simulink model "variant1"  (R2018a)
settings: Solver=VariableStepAuto  StartTime=0.0  StopTime=10.0  RelTol=1e-3
undefined symbols (not defined in the file or in its folder): gray
libraries: simulink x4, visionstatistics x2, visiontransforms x1
settings Model: Creator=Farwa  LastModifiedBy=Farwa

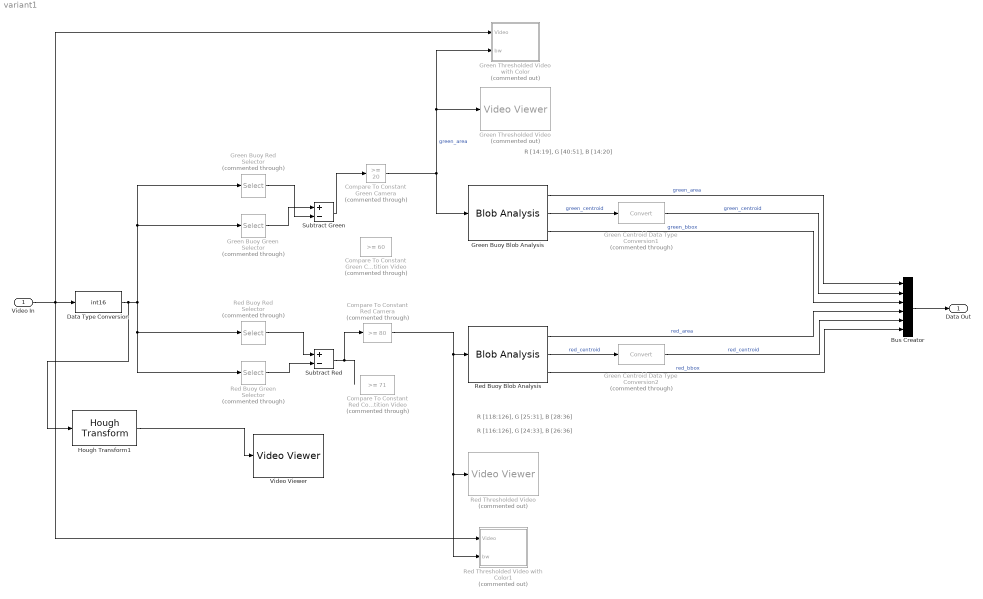
== system variant1 ==
  note: R [118:126], G [25:31], B [28:36]
  note: R [116:126], G [24:33], B [26:36]
  note: R [14:19], G [40:51], B [14:20]
  Video In : Inport
  Bus Creator : BusCreator  Inputs=6
  Compare To Constant Green Camera : simulink/Logic and Bit Operations/Compare To Constant  Commented=through  relop=>=  const=20  OutDataTypeStr=boolean
  Compare To Constant Green Competition Video : simulink/Logic and Bit Operations/Compare To Constant  Commented=through  relop=>=  const=60  OutDataTypeStr=boolean
  Compare To Constant Red Camera : simulink/Logic and Bit Operations/Compare To Constant  Commented=through  relop=>=  const=80  OutDataTypeStr=boolean
  Compare To Constant Red Competition Video : simulink/Logic and Bit Operations/Compare To Constant  Commented=through  relop=>=  const=71  OutDataTypeStr=boolean
  Data Type Conversion : DataTypeConversion  OutDataTypeStr=int16
  Green Buoy Blob Analysis : visionstatistics/Blob Analysis  Tag=vipblks_row_conv  area=on  centroid=on  bBox=on  majorAxis=off  minorAxis=off  angle=off  eccentricity=off  equivDiameterSq=off  extent=off  perimeter=off  maxBlobs=4  warnIfNumBlobsExceeded=off  isCount=off  useMinArea=on  minArea=40  useMaxArea=off  maxArea=100  excludeBorderBlob=off  outDT=single  isOutVarDim=off  isFill=on  fillValues=-1  conn=8  isLabel=off  outputMode=Binary point scaling  outputWordLength=32  outputFracLength=16  firstCoeffMode=Binary point scaling  firstCoeffWordLength=16  firstCoeffFracLength=14  secondCoeffMode=Binary point scaling  secondCoeffWordLength=32  secondCoeffFracLength=16  accumMode=Binary point scaling  accumWordLength=32  accumFracLength=0  prodOutputMode=Binary point scaling  prodOutputWordLength=32  prodOutputFracLength=16  roundingMode=Floor  overflowMode=off
      settings: SourceProductName=Computer Vision System Toolbox
  Green Buoy Green Selector : Selector  Commented=through  NumberOfDimensions=3  InputPortWidth=3  IndexOptions=Select all,Select all,Index vector (dialog)  Indices=[1 3],1,2  OutputSizes=1,1,1
  Green Buoy Red Selector : Selector  Commented=through  NumberOfDimensions=3  InputPortWidth=3  IndexOptions=Select all,Select all,Index vector (dialog)  Indices=[1 3],1,1  OutputSizes=1,1,1
  Green Centroid Data Type Conversion1 : DataTypeConversion  Commented=through
  Green Centroid Data Type Conversion2 : DataTypeConversion  Commented=through
  Green Thresholded Video : VideoViewer  Commented=on  colormapValue=gray(256)  FigPos=[1107 745 758 524]
  Green Thresholded Video with Color : Subsystem  Commented=on
  Hough Transform1 : visiontransforms/Hough Transform  theta_res=pi/180  rho_res=1  out_theta_rho=off  outdtmode=double  firstCoeffMode=Binary point scaling  firstCoeffWordLength=16  firstCoeffFracLength=14  secondCoeffMode=Binary point scaling  secondCoeffWordLength=32  secondCoeffFracLength=16  outputMode=Binary point scaling  outputWordLength=16  outputFracLength=0  accumMode=Binary point scaling  accumWordLength=32  accumFracLength=20  prodOutputMode=Binary point scaling  prodOutputWordLength=32  prodOutputFracLength=20  memoryMode=Binary point scaling  memoryWordLength=32  memoryFracLength=16  roundingMode=Nearest  overflowMode=on
      settings: SourceProductName=Computer Vision System Toolbox  SourceProductBaseCode=VP
  Red Buoy Blob Analysis : visionstatistics/Blob Analysis  Tag=vipblks_row_conv  area=on  centroid=on  bBox=on  majorAxis=off  minorAxis=off  angle=off  eccentricity=off  equivDiameterSq=off  extent=off  perimeter=off  maxBlobs=4  warnIfNumBlobsExceeded=off  isCount=off  useMinArea=on  minArea=20  useMaxArea=off  maxArea=100  excludeBorderBlob=off  outDT=double  isOutVarDim=off  isFill=on  fillValues=-1  conn=8  isLabel=off  outputMode=Binary point scaling  outputWordLength=32  outputFracLength=16  firstCoeffMode=Binary point scaling  firstCoeffWordLength=16  firstCoeffFracLength=14  secondCoeffMode=Binary point scaling  secondCoeffWordLength=32  secondCoeffFracLength=16  accumMode=Binary point scaling  accumWordLength=32  accumFracLength=0  prodOutputMode=Binary point scaling  prodOutputWordLength=32  prodOutputFracLength=16  roundingMode=Floor  overflowMode=off
      settings: SourceProductName=Computer Vision System Toolbox
  Red Buoy Green Selector : Selector  Commented=through  NumberOfDimensions=3  InputPortWidth=3  IndexOptions=Select all,Select all,Index vector (dialog)  Indices=[1 3],1,2  OutputSizes=1,1,1
  Red Buoy Red Selector : Selector  Commented=through  NumberOfDimensions=3  InputPortWidth=3  IndexOptions=Select all,Select all,Index vector (dialog)  Indices=[1 3],1,1  OutputSizes=1,1,1
  Red Thresholded Video : VideoViewer  Commented=on  colormapValue=gray(256)  FigPos=[1008 1320 758 524]
  Red Thresholded Video with Color1 : Subsystem  Commented=on
  Subtract Green : Sum  Inputs=+-  OutDataTypeStr=Inherit: Same as first input
  Subtract Red : Sum  Inputs=+-  OutDataTypeStr=Inherit: Same as first input
  Video Viewer : VideoViewer  FigPos=[431 511 418 304]
  Data Out : Outport
  wires:
  Green Buoy Blob Analysis/2 -> Green Centroid Data Type Conversion1/1  "green_centroid"
  Green Centroid Data Type Conversion1/1 -> Bus Creator/2  "green_centroid"
  Red Buoy Blob Analysis/1 -> Bus Creator/4  "red_area"
  Bus Creator/1 -> Data Out/1
  Red Buoy Green Selector/1 -> Subtract Red/2
  Green Buoy Blob Analysis/3 -> Bus Creator/3  "green_bbox"
  Red Buoy Blob Analysis/3 -> Bus Creator/6  "red_bbox"
  Compare To Constant Green Camera/1 -> Green Buoy Blob Analysis/1, Green Thresholded Video with Color/2(bw), Green Thresholded Video/1  "green_area"
  Subtract Green/1 -> Compare To Constant Green Camera/1
  Video In/1 -> Data Type Conversion/1, Green Thresholded Video with Color/1(Video), Red Thresholded Video with Color1/1(Video)
  Green Buoy Blob Analysis/1 -> Bus Creator/1  "green_area"
  Green Buoy Green Selector/1 -> Subtract Green/1
  Hough Transform1/1 -> Video Viewer/1
  Green Buoy Red Selector/1 -> Subtract Green/2
  Red Buoy Blob Analysis/2 -> Green Centroid Data Type Conversion2/1  "red_centroid"
  Red Buoy Red Selector/1 -> Subtract Red/1
  Data Type Conversion/1 -> Hough Transform1/1, Red Buoy Green Selector/1, Red Buoy Red Selector/1, Green Buoy Red Selector/1, Green Buoy Green Selector/1
  Green Centroid Data Type Conversion2/1 -> Bus Creator/5  "red_centroid"
  Compare To Constant Red Camera/1 -> Red Thresholded Video with Color1/2(bw), Red Thresholded Video/1, Red Buoy Blob Analysis/1
  Subtract Red/1 -> Compare To Constant Red Camera/1

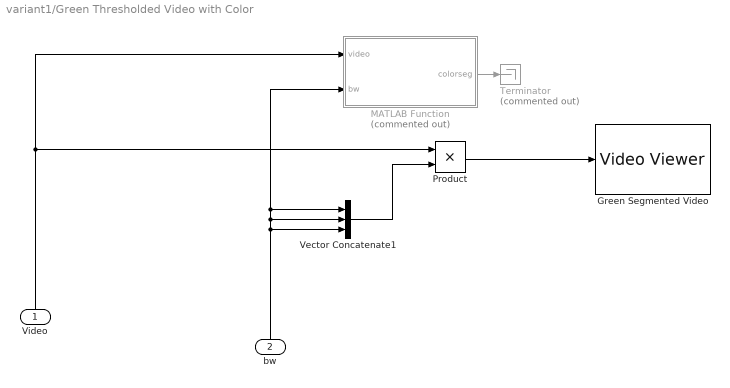
== system variant1/Green Thresholded Video with Color ==
  Video : Inport
  bw : Inport  Port=2
  "Green Segmented Video " : VideoViewer  colormapValue=gray(256)  FigPos=[1034 644 758 524]
  MATLAB Function : MATLAB Function  Commented=on  TreatAsAtomicUnit=on
  Product : Product
  Terminator : Terminator  Commented=on
  Vector Concatenate1 : Concatenate  NumInputs=3  Mode=Multidimensional array  ConcatenateDimension=3
  wires:
  bw/1 -> MATLAB Function/2(bw), Vector Concatenate1/1, Vector Concatenate1/2, Vector Concatenate1/3
  MATLAB Function/1(colorseg) -> Terminator/1
  Video/1 -> Product/1, MATLAB Function/1(video)
  Product/1 -> "Green Segmented Video "/1
  Vector Concatenate1/1 -> Product/2

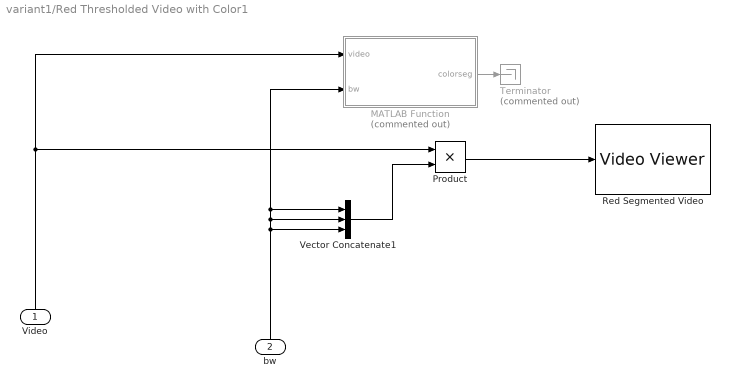
== system variant1/Red Thresholded Video with Color1 ==
  Video : Inport
  bw : Inport  Port=2
  MATLAB Function : MATLAB Function  Commented=on  TreatAsAtomicUnit=on
  Product : Product
  "Red Segmented Video " : VideoViewer  colormapValue=gray(256)  FigPos=[423.666666666667 763.333333333333 758 524]
  Terminator : Terminator  Commented=on
  Vector Concatenate1 : Concatenate  NumInputs=3  Mode=Multidimensional array  ConcatenateDimension=3
  wires:
  bw/1 -> MATLAB Function/2(bw), Vector Concatenate1/1, Vector Concatenate1/2, Vector Concatenate1/3
  MATLAB Function/1(colorseg) -> Terminator/1
  Video/1 -> Product/1, MATLAB Function/1(video)
  Product/1 -> "Red Segmented Video "/1
  Vector Concatenate1/1 -> Product/2

== matlab function variant1/Green Thresholded Video with Color/MATLAB Function ==
  data: video input; colorseg output; bw input
function colorseg = fcn(video,bw)
%#codegen

% overlay color onto thresholded bw image
% can be used to clean up noise easily
% comment out if unnecessary
colorseg = uint8(repmat(bw,[1,1,3]).*double(video));

== matlab function variant1/Red Thresholded Video with Color1/MATLAB Function ==
  data: video input; colorseg output; bw input
function colorseg = fcn(video,bw)
%#codegen

% overlay color onto thresholded bw image
% can be used to clean up noise easily
% comment out if unnecessary
colorseg = uint8(repmat(bw,[1,1,3]).*double(video));
